simulink model "function2"  (R2019a)
settings: Solver=VariableStepAuto  StartTime=0.0  StopTime=2000  RelTol=1e-3
undefined symbols (not defined in the file): Ion, Lithium
libraries: powerlib x14, electricdrivelib x3
settings Model: SimulationMode=accelerator  Creator=rachad  LastModifiedBy=رشاد
settings SolverCC: ZeroCrossAlgorithm=Adaptive
settings DebuggingCC: IgnoredZcDiagnostic=none

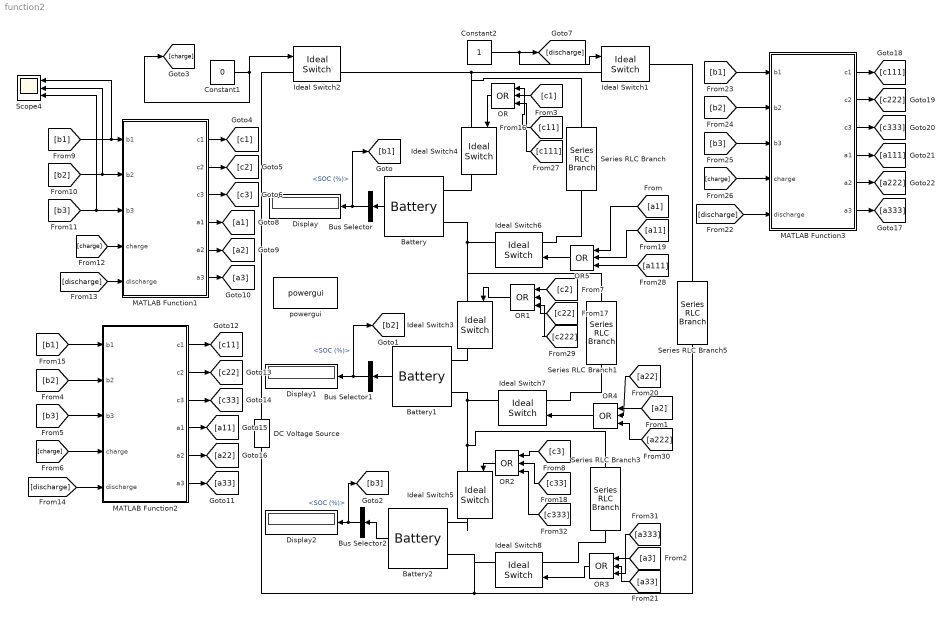
== system function2 ==
  Battery : electricdrivelib/Extra Sources/Battery  BatType=Lithium-Ion  ShowTempParam=off  ThermalPreset=no  ShowAgeParam=off  NomV=3.6  NomQ=2.6  SOC=100  Batt_Tr=3  PresetModel=on  MaxQ=2.6  MinV=2.7  FullV=4.1904  Dis_rate=1.1304  R=0.013846  Normal_OP=2.3513  expZone="[3.8894     0.12774]"  current=[6.5 13 32.5]  Units=Time  Tci=20  NomT=20  T2=-30  MaxQ2=4.8  FullV2=7.1  Normal_OP2=5.655  expZone2="[6.58           1]"  Rca=0.6  ti=2000  Dp=0  Neq0=0  Tsim=1e6  Ta1=25  Qeol=5.4*0.9  Reol=0.013333*1.2  Char_age=[2.3478, 3]  Dis_age=[2.3478, 10]  N1=1500  N2=10500  N3=1000  N4=1400  Ta2=45  N5=950
      settings: SourceProductName=Simscape Electrical
  Battery1 : electricdrivelib/Extra Sources/Battery  BatType=Lithium-Ion  ShowTempParam=off  ThermalPreset=no  ShowAgeParam=off  NomV=3.6  NomQ=2.6  SOC=90  Batt_Tr=3  PresetModel=on  MaxQ=2.6  MinV=2.7  FullV=4.1904  Dis_rate=1.1304  R=0.013846  Normal_OP=2.3513  expZone="[3.8894     0.12774]"  current=[6.5 13 32.5]  Units=Time  Tci=20  NomT=20  T2=-30  MaxQ2=4.8  FullV2=7.1  Normal_OP2=5.655  expZone2="[6.58           1]"  Rca=0.6  ti=2000  Dp=0  Neq0=0  Tsim=1e6  Ta1=25  Qeol=5.4*0.9  Reol=0.013333*1.2  Char_age=[2.3478, 3]  Dis_age=[2.3478, 10]  N1=1500  N2=10500  N3=1000  N4=1400  Ta2=45  N5=950
      settings: SourceProductName=Simscape Electrical
  Battery2 : electricdrivelib/Extra Sources/Battery  BatType=Lithium-Ion  ShowTempParam=off  ThermalPreset=no  ShowAgeParam=off  NomV=3.6  NomQ=2.6  SOC=18  Batt_Tr=3  PresetModel=on  MaxQ=2.6  MinV=2.7  FullV=4.1904  Dis_rate=1.1304  R=0.013846  Normal_OP=2.3513  expZone="[3.8894     0.12774]"  current=[6.5 13 32.5]  Units=Time  Tci=20  NomT=20  T2=-30  MaxQ2=4.8  FullV2=7.1  Normal_OP2=5.655  expZone2="[6.58           1]"  Rca=0.6  ti=2000  Dp=0  Neq0=0  Tsim=1e6  Ta1=25  Qeol=5.4*0.9  Reol=0.013333*1.2  Char_age=[2.3478, 3]  Dis_age=[2.3478, 10]  N1=1500  N2=10500  N3=1000  N4=1400  Ta2=45  N5=950
      settings: SourceProductName=Simscape Electrical
  Bus Selector : BusSelector  OutputSignals=SOC (%)
  Bus Selector1 : BusSelector  OutputSignals=SOC (%)
  Bus Selector2 : BusSelector  OutputSignals=SOC (%)
  Constant1 : Constant  Value=0
  Constant2 : Constant
  DC Voltage Source : powerlib/Electrical Sources/DC Voltage Source  Amplitude=25  Measurements=None
      settings: SourceProductName=Simscape Electrical
  Display : Display
  Display1 : Display
  Display2 : Display
  Ideal Switch1 : powerlib/Power Electronics/Ideal Switch  Ron=0.001  Lon=0  IC=0  Rs=inf  Cs=inf  Measurements=off
      settings: SourceProductName=Simscape Electrical
  Ideal Switch{2..8} (7 alike) : powerlib/Power Electronics/Ideal Switch  Ron=0.001  Lon=0  IC=0  Rs=inf  Cs=inf  Measurements=on
      settings: SourceProductName=Simscape Electrical
  MATLAB Function1 : MATLAB Function  TreatAsAtomicUnit=on
  MATLAB Function2 : MATLAB Function  TreatAsAtomicUnit=on
  MATLAB Function3 : MATLAB Function  TreatAsAtomicUnit=on
  OR{,1..5} (6 alike) : Logic  Operator=OR  Inputs=3  IconShape=distinctive  AllPortsSameDT=off  OutDataTypeStr=boolean
  Scope4 : Scope  NumInputPorts=3
  Series RLC Branch : powerlib/Elements/Series RLC Branch  LConnTagsString=__new0  RConnTagsString=__new0  BranchType=R  Resistance=1  Inductance=1e-3  SetiL0=off  InitialCurrent=0  Capacitance=1e-6  Setx0=off  InitialVoltage=0  Measurements=None
      settings: SourceProductName=Simscape Electrical
  Series RLC Branch1 : powerlib/Elements/Series RLC Branch  LConnTagsString=__new0  RConnTagsString=__new0  BranchType=R  Resistance=1  Inductance=1e-3  SetiL0=off  InitialCurrent=0  Capacitance=1e-6  Setx0=off  InitialVoltage=0  Measurements=None
      settings: SourceProductName=Simscape Electrical
  Series RLC Branch3 : powerlib/Elements/Series RLC Branch  LConnTagsString=__new0  RConnTagsString=__new0  BranchType=R  Resistance=1  Inductance=1e-3  SetiL0=off  InitialCurrent=0  Capacitance=1e-6  Setx0=off  InitialVoltage=0  Measurements=None
      settings: SourceProductName=Simscape Electrical
  Series RLC Branch5 : powerlib/Elements/Series RLC Branch  LConnTagsString=__new0  RConnTagsString=__new0  BranchType=R  Resistance=0.0001  Inductance=1e-3  SetiL0=off  InitialCurrent=0  Capacitance=1e-6  Setx0=off  InitialVoltage=0  Measurements=None
      settings: SourceProductName=Simscape Electrical
  powergui : powerlib/powergui  Priority=1  SimulationMode=Continuous  SampleTime=50e-6  frequency=60  Iterations=50  frequencyindice=0  Pbase=100e6  ErrMax=1e-4  UnitsV=kV  UnitsW=MW  buscounter=0  FunctionMessages=off  echomessages=off  EnableUseOfTLC=off  CurrentSourceSwitches=off  DisableSnubberDevices=off  DisableRonSwitches=off  DisableVfSwitches=off  DisplayEquations=off  AutomaticDiscreteSolvers=off  SolverType=Tustin/Backward Euler (TBE)  Interpol=off  ExternalGateDelay=off  methode=off  Ts=100  x0status=blocks  SPID=on  SwTol=0  HookPort=off  NonlinearTolerance=0  nMaxIteration=15  ContinueOnMaxIteration=off  RestoreLinks=warning  ResistiveCurrentMeasurement=off  Frange=[0:2:500]  Ylog=off  Xlog=on  ShowGrid=off  save=off  variable=ZData  structure=0  ZoomFFT=off  StartTime=0.0  cycles=1  DisplayStyle=1  fundamental=60  FreqAxis=off  MaxFrequency=1000  frequencyindicesteady=1  RmsSteady=1  display=off
      settings: SourceProductName=Simscape Electrical
  wires:
  Battery/1 -> Bus Selector/1
  Battery1/1 -> Bus Selector1/1
  Battery2/1 -> Bus Selector2/1
  Bus Selector/1 -> [b1], Display/1  "<SOC (%)>"
  Constant1/1 -> Ideal Switch2/1, [charge]
  Constant2/1 -> Ideal Switch1/1, [discharge]
  Bus Selector2/1 -> [b3], Display2/1  "<SOC (%)>"
  Bus Selector1/1 -> Display1/1, [b2]  "<SOC (%)>"
  MATLAB Function1/4(a1) -> [a1]
  MATLAB Function1/5(a2) -> [a2]
  MATLAB Function1/6(a3) -> [a3]
  [b1] -> Scope4/1, MATLAB Function1/1(b1)
  [b2] -> Scope4/2, MATLAB Function1/2(b2)
  [b3] -> Scope4/3, MATLAB Function1/3(b3)
  [charge] -> MATLAB Function1/4(charge)
  [discharge] -> MATLAB Function1/5(discharge)
  MATLAB Function1/1(c1) -> [c1]
  MATLAB Function1/2(c2) -> [c2]
  MATLAB Function1/3(c3) -> [c3]
  MATLAB Function2/3(c3) -> [c33]
  MATLAB Function2/2(c2) -> [c22]
  MATLAB Function2/1(c1) -> [c11]
  [discharge] -> MATLAB Function2/5(discharge)
  [charge] -> MATLAB Function2/4(charge)
  [b3] -> MATLAB Function2/3(b3)
  [b2] -> MATLAB Function2/2(b2)
  [b1] -> MATLAB Function2/1(b1)
  MATLAB Function2/6(a3) -> [a33]
  MATLAB Function2/5(a2) -> [a22]
  MATLAB Function2/4(a1) -> [a11]
  OR/1 -> Ideal Switch4/1
  [c1] -> OR/1
  [c11] -> OR/2
  [c2] -> OR1/1
  [c22] -> OR1/2
  OR1/1 -> Ideal Switch3/1
  OR2/1 -> Ideal Switch5/1
  [c3] -> OR2/1
  [c33] -> OR2/2
  [a1] -> OR5/1
  [a11] -> OR5/2
  [a2] -> OR4/1
  [a22] -> OR4/2
  [a3] -> OR3/1
  [a33] -> OR3/2
  MATLAB Function3/4(a1) -> [a111]
  MATLAB Function3/5(a2) -> [a222]
  MATLAB Function3/6(a3) -> [a333]
  [b1] -> MATLAB Function3/1(b1)
  [b2] -> MATLAB Function3/2(b2)
  [b3] -> MATLAB Function3/3(b3)
  [charge] -> MATLAB Function3/4(charge)
  [discharge] -> MATLAB Function3/5(discharge)
  MATLAB Function3/1(c1) -> [c111]
  MATLAB Function3/2(c2) -> [c222]
  MATLAB Function3/3(c3) -> [c333]
  [c111] -> OR/3
  [a111] -> OR5/3
  [c222] -> OR1/3
  [a222] -> OR4/3
  [a333] -> OR3/3
  [c333] -> OR2/3
  OR5/1 -> Ideal Switch6/1
  OR4/1 -> Ideal Switch7/1
  OR3/1 -> Ideal Switch8/1
  connections:
  Battery/LConn2 -- Ideal Switch3/LConn1 -- Series RLC Branch1/LConn1 -- Ideal Switch6/RConn1
  Battery1/LConn2 -- Series RLC Branch3/LConn1 -- Ideal Switch5/LConn1 -- Ideal Switch7/RConn1
  Ideal Switch1/LConn1 -- Ideal Switch4/LConn1 -- Series RLC Branch/LConn1 -- Ideal Switch2/RConn1
  DC Voltage Source/LConn1 -- Ideal Switch8/RConn1 -- Battery2/LConn2 -- Series RLC Branch5/RConn1
  Series RLC Branch5/LConn1 -- Ideal Switch1/RConn1
  Ideal Switch2/LConn1 -- DC Voltage Source/RConn1
  Ideal Switch5/RConn1 -- Battery2/LConn1
  Ideal Switch4/RConn1 -- Battery/LConn1
  Ideal Switch3/RConn1 -- Battery1/LConn1
  Ideal Switch6/LConn1 -- Series RLC Branch/RConn1
  Ideal Switch7/LConn1 -- Series RLC Branch1/RConn1
  Series RLC Branch3/RConn1 -- Ideal Switch8/LConn1

== matlab function function2/MATLAB Function1 ==
  data: c1 output; b1 input; b2 input; b3 input; charge input; c2 output; c3 output; discharge input; a1 output; a2 output; a3 output
function [c1, c2, c3,a1,a2,a3]= fcn(b1, b2, b3, charge, discharge)
b1=b1*100;
b2=b2*100;
b3=b3*100;
b1=int32(b1);
b2=int32(b2);
b3=int32(b3);
if discharge==0 && charge==0 
    if b1==b2 && b2==b3
    a1=0;
    a2=0;
    a3=0;
    c1=0;
    c2=0;
    c3=0;
    elseif max([b1 b2 b3])== b1
    a1=1;
    a2=0;
    a3=0;
    c1=1;c2=1;c3=1;
    elseif max([b1 b2 b3])== b2
    a2=1;
    a1=0;
    a3=0;
    c1=1;c2=1;c3=1; 
elseif max([b1 b2 b3])== b3
    a3=1;
    a1=0;
    a2=0;
    c1=1;c2=1;c3=1;   
    else
    a1=0;
    a2=0;
   a3=0;
    c1=1;
    c2=1;
    c3=1;
    end        
else
    a1=0;
    a2=0;
    a3=0;
    c1=0;
    c2=0;
    c3=0;  
end 
end

== matlab function function2/MATLAB Function2 ==
  data: c1 output; b1 input; b2 input; b3 input; charge input; c2 output; c3 output; discharge input; a1 output; a2 output; a3 output
function [c1, c2, c3,a1,a2,a3]= fcn(b1, b2, b3, charge, discharge)
b1=b1*1;
b2=b2*1;
b3=b3*1;
b1=int32(b1);
b2=int32(b2);
b3=int32(b3);
if discharge==0 && charge==1 
     if b1<=90 || b2<=90 || b3<=90   
     if b2<=90  
    a1=1;
    a2=0;
    a3=1;
    c1=0;
    c2=1;
    c3=0;
    else
    a1=1;
    a2=1;
    a3=1;
    c1=0;
    c2=0;
    c3=0;
     end 
       if b3<=90   
          if b1<=90 
          if b2<=90  
    a1=0;
    a2=0;
    a3=0;
    c1=1;
    c2=1;
    c3=1;
    else
    a1=0;
    a2=1;
    a3=0;
    c1=1;
    c2=0;
    c3=1;
     end    
          else
        if b2<=90  
    a1=1;
    a2=0;
    a3=0;
    c1=0;
    c2=1;
    c3=1;
    else
    a1=1;
    a2=1;
    a3=0;
    c1=0;
    c2=0;
    c3=1;
     end 
          end  
       else    
       if b1<=90  
          if b2<=90  
    a1=0;
    a2=0;
    a3=1;
    c1=1;
    c2=1;
    c3=0;
    else
    a1=0;
    a2=1;
    a3=1;
    c1=1;
    c2=0;
    c3=0;
     end  
       else
      if b2<=90  
    a1=1;
    a2=0;
    a3=1;
    c1=0;
    c2=1;
    c3=0;
    else
    a1=1;
    a2=1;
    a3=1;
    c1=0;
    c2=0;
    c3=0;
     end       
        end 
       end 
     else
    a3=0;
    a1=0;
    a2=0;
    c1=1;
    c2=1;
    c3=1;  
     end 
   else
    a1=0;
    a2=0;
    a3=0;
    c1=0;
    c2=0;
    c3=0;
end
end

== matlab function function2/MATLAB Function3 ==
  data: c1 output; b1 input; b2 input; b3 input; charge input; c2 output; c3 output; discharge input; a1 output; a2 output; a3 output
function [c1, c2, c3,a1,a2,a3]= fcn(b1, b2, b3, charge, discharge)
b1=b1*1;
b2=b2*1;
b3=b3*1;
b1=int32(b1);
b2=int32(b2);
b3=int32(b3);
if discharge==1 && charge==0 
     if b1>=15 || b2>=15 || b3>=15  
  if b1>15
      if b2>15
          if b3>15
    a1=0;
    a2=0;
    a3=0;
    c1=1;
    c2=1;
    c3=1;
          else
    a1=0;
    a2=0;
    a3=1;
    c1=1;
    c2=1;
    c3=0;    
          end
      else
          if b3> 15
    a1=0;
    a2=1;
    a3=0;
    c1=1;
    c2=0;
    c3=1; 
          else
    a1=0;
    a2=1;
    a3=1;
    c1=1;
    c2=0;
    c3=0; 
          end
      end
  else
      if b2>15
          if b3>15
    a1=1;
    a2=0;
    a3=0;
    c1=0;
    c2=1;
    c3=1;    
          else
    a1=1;
    a2=0;
    a3=1;
    c1=0;
    c2=1;
    c3=0;  
          end
      else
          if b3>15
    a1=1;
    a2=1;
    a3=0;
    c1=0;
    c2=0;
    c3=1;   
          else 
    a1=1;
    a2=1;
    a3=1;
    c1=0;
    c2=0;
    c3=0;  
          end
      end
  end    
   else
    a1=0;
    a2=0;
    a3=0;
    c1=0;
    c2=0;
    c3=0;
     end
else
   a1=0;
    a2=0;
    a3=0;
    c1=0;
    c2=0;
    c3=0; 
end
end
